simulink model "Sim21"  (R2019a)
settings: Solver=VariableStepAuto  StartTime=0.0  StopTime=10.0  RelTol=1e-3
settings Model: Creator=fbleo  LastModifiedBy=fbleo

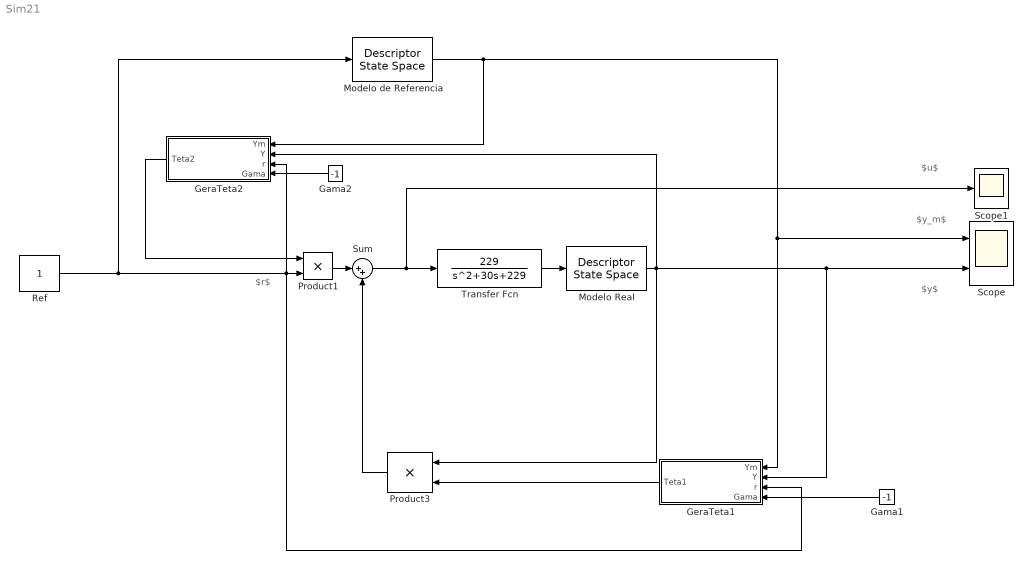
== system Sim21 ==
  note: $y$
  note: $u$
  note: $r$
  note: $y_m$
  Gama1 : Constant  Value=-1
  Gama2 : Constant  Value=-1
  GeraTeta1 : Subsystem
  GeraTeta2 : Subsystem
  Modelo Real : DescriptorStateSpace  A=-1  B=2  D=0  InitialCondition=0.5
  Modelo de Referencia : DescriptorStateSpace  A=-3  B=3  D=0  InitialCondition=0
  Product1 : Product
  Product3 : Product
  Ref : Constant
  Scope : Scope  NumInputPorts=2
  Scope1 : Scope
  Sum : Sum  Inputs=|++
  Transfer Fcn : TransferFcn  Numerator=[229]  Denominator=[1 30 229]
  wires:
  Modelo Real/1 -> GeraTeta2/2(Y), GeraTeta1/2(Y), Scope/2, Product3/1
  Product1/1 -> Sum/1
  Sum/1 -> Scope1/1, Transfer Fcn/1
  GeraTeta1/1("Teta1 ") -> Product3/2
  GeraTeta2/1(Teta2) -> Product1/1
  Product3/1 -> Sum/2
  Transfer Fcn/1 -> Modelo Real/1
  Modelo de Referencia/1 -> GeraTeta2/1(Ym), GeraTeta1/1(Ym), Scope/1
  Gama2/1 -> GeraTeta2/4(Gama)
  Gama1/1 -> GeraTeta1/4(Gama)
  Ref/1 -> GeraTeta1/3(r), GeraTeta2/3(r), Product1/2, Modelo de Referencia/1

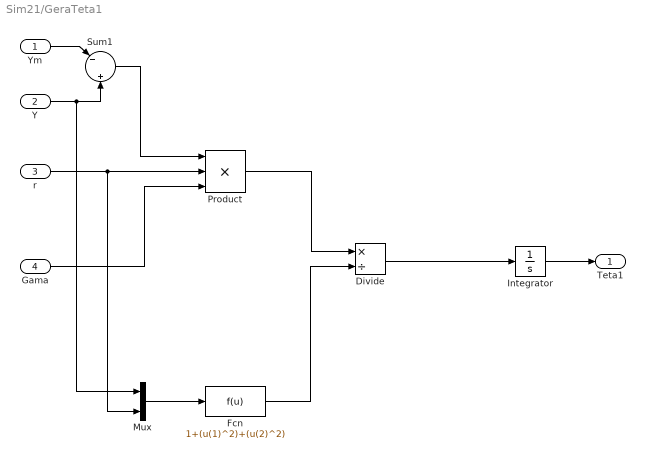
== system Sim21/GeraTeta1 ==
  Ym : Inport
  Y : Inport  Port=2
  r : Inport  Port=3
  Gama : Inport  Port=4
  Divide : Product  Inputs=*/
  Fcn : Fcn  Expr=1+(u(1)^2)+(u(2)^2)
  Integrator : Integrator  InitialCondition=-0.65
  Mux : Mux  Inputs=2
  Product : Product  Inputs=3
  Sum1 : Sum  Inputs=|-||+
  "Teta1 " : Outport
  wires:
  Ym/1 -> Sum1/1
  Y/1 -> Mux/1, Sum1/2
  Sum1/1 -> Product/1
  r/1 -> Mux/2, Product/2
  Gama/1 -> Product/3
  Integrator/1 -> "Teta1 "/1
  Mux/1 -> Fcn/1
  Product/1 -> Divide/1
  Fcn/1 -> Divide/2
  Divide/1 -> Integrator/1

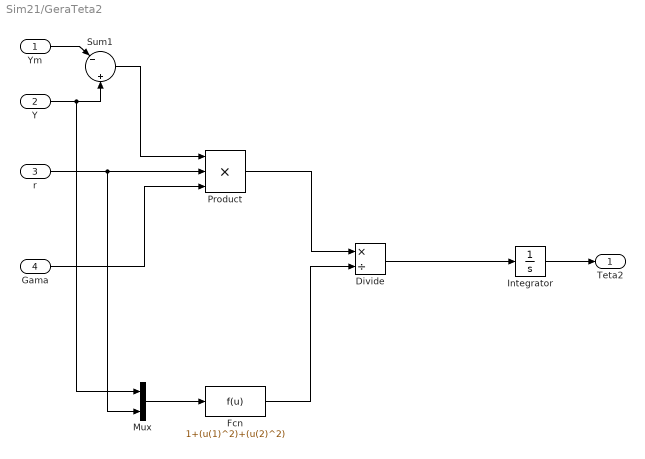
== system Sim21/GeraTeta2 ==
  Ym : Inport
  Y : Inport  Port=2
  r : Inport  Port=3
  Gama : Inport  Port=4
  Divide : Product  Inputs=*/
  Fcn : Fcn  Expr=1+(u(1)^2)+(u(2)^2)
  Integrator : Integrator  InitialCondition=1.14
  Mux : Mux  Inputs=2
  Product : Product  Inputs=3
  Sum1 : Sum  Inputs=|-||+
  Teta2 : Outport
  wires:
  Ym/1 -> Sum1/1
  Y/1 -> Mux/1, Sum1/2
  Sum1/1 -> Product/1
  r/1 -> Mux/2, Product/2
  Gama/1 -> Product/3
  Integrator/1 -> Teta2/1
  Mux/1 -> Fcn/1
  Product/1 -> Divide/1
  Fcn/1 -> Divide/2
  Divide/1 -> Integrator/1
